simulink model "deteccion_prueba"  (R2018a)
settings: Solver=VariableStepAuto  StartTime=0.0  StopTime=0.8  RelTol=1e-3
values from neighbouring files (symbols this model uses):
  tm = 1e-4    (= 0.0001)    [SimulinkInit.m]
settings Model: Creator=cmparedes  LastModifiedBy=cmparedes

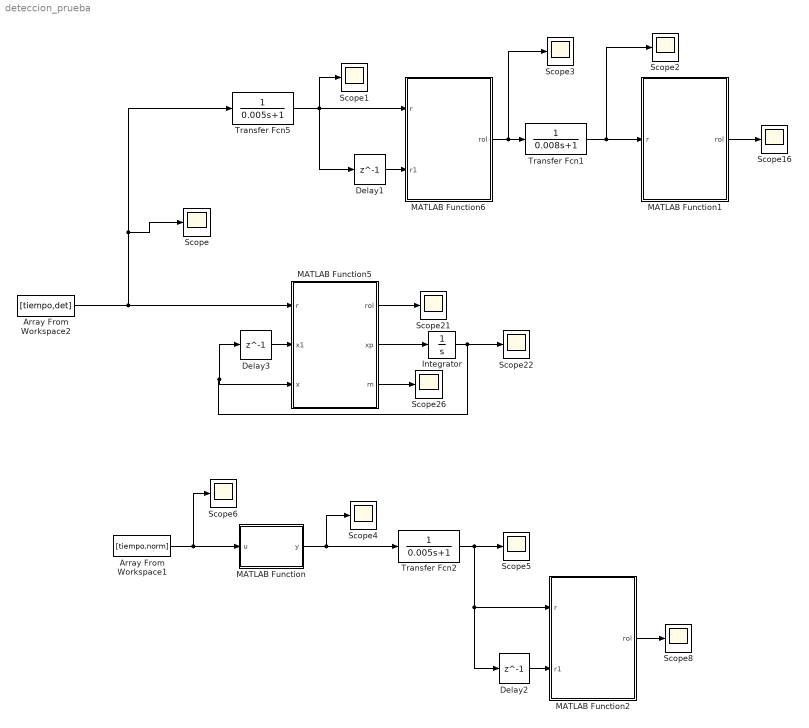
== system deteccion_prueba ==
  Array From Workspace1 : FromWorkspace  VariableName=[tiempo,norm]  SampleTime=tm
  Array From Workspace2 : FromWorkspace  VariableName=[tiempo,det]  SampleTime=tm
  Delay1 : Delay  DelayLength=1
  Delay2 : Delay  DelayLength=1
  Delay3 : Delay  DelayLength=1
  Integrator : Integrator
  MATLAB Function : MATLAB Function  TreatAsAtomicUnit=on
  MATLAB Function1 : MATLAB Function  TreatAsAtomicUnit=on
  MATLAB Function2 : MATLAB Function  TreatAsAtomicUnit=on
  MATLAB Function5 : MATLAB Function  TreatAsAtomicUnit=on
  MATLAB Function6 : MATLAB Function  TreatAsAtomicUnit=on
  Scope{,1..6,8,16,21..22,26} (12 alike) : Scope
  Transfer Fcn1 : TransferFcn  Denominator=[0.008 1]
  Transfer Fcn2 : TransferFcn  Denominator=[0.005 1]
  Transfer Fcn5 : TransferFcn  Denominator=[0.005 1]
  wires:
  MATLAB Function5/3(m) -> Scope26/1
  MATLAB Function5/1(rol) -> Scope21/1
  MATLAB Function5/2(xp) -> Integrator/1
  Integrator/1 -> Delay3/1, MATLAB Function5/3(x), Scope22/1
  MATLAB Function6/1(rol) -> Scope3/1, Transfer Fcn1/1
  Delay1/1 -> MATLAB Function6/2(r1)
  Transfer Fcn5/1 -> Scope1/1, MATLAB Function6/1(r), Delay1/1
  Array From Workspace2/1 -> Scope/1, Transfer Fcn5/1, MATLAB Function5/1(r)
  Delay3/1 -> MATLAB Function5/2(x1)
  Transfer Fcn1/1 -> Scope2/1, MATLAB Function1/1(r)
  MATLAB Function1/1(rol) -> Scope16/1
  Array From Workspace1/1 -> Scope6/1, MATLAB Function/1(u)
  Transfer Fcn2/1 -> Delay2/1, MATLAB Function2/1(r), Scope5/1
  MATLAB Function/1(y) -> Transfer Fcn2/1, Scope4/1
  Delay2/1 -> MATLAB Function2/2(r1)
  MATLAB Function2/1(rol) -> Scope8/1

== matlab function deteccion_prueba/MATLAB Function1 ==
  data: r input; rol output
function rol = fcn(r)%u1,u2,ym1,ym2)
Th_det = 6.5e-8;
% Th_det=0.1;  %2.5

if r >=Th_det
    rol=1;
else
    rol=0;
end

== matlab function deteccion_prueba/MATLAB Function ==
  data: u input; y output
function y = fcn(u)

if u>0.07

    y = 1;
else
    y=0;
end

== matlab function deteccion_prueba/MATLAB Function2 ==
  data: r input; rol output; r1 input
function rol = fcn(r,r1)%u1,u2,ym1,ym2)
Th_det = 6.5e-8;
Th_det=0.1;  %2.5

m=r-r1;
if m>0
    Th_det=0.1;  %2.5
elseif m<0 && r<=0.01
    Th_det=0.9; 
end


% sys=tf(1,[0.001 1]);


if r >=Th_det
    rol=1;
else
    rol=0;
end

== matlab function deteccion_prueba/MATLAB Function5 ==
  data: r input; rol output; x1 input; xp output; x input; m output
function [rol,xp,m]= fcn(r,x1,x)%u1,u2,ym1,ym2)
Th_det = 6.5e-8;
Th_det=0.1;  %2.5

tao1=0.002;
tao2=0.02;
m=x-x1;

xp= r/tao1-x/tao1;

% xp=0;

if m>0
    xp= r/tao1-x/tao1;
    Th_det=0.1;  %2.5
elseif m<0 && x<=-1
    xp= r/tao2-x/tao2;
    Th_det=0.08; 
end



% sys=tf(1,[0.001 1]);


if x >=Th_det
    rol=1;
else
    rol=0;
end

== matlab function deteccion_prueba/MATLAB Function6 ==
  data: r input; rol output; r1 input
function rol = fcn(r,r1)%u1,u2,ym1,ym2)
Th_det = 6.5e-8;
Th_det=0.1;  %2.5

m=r-r1;
if m>0
    Th_det=0.1;  %2.5
elseif m<0 && r<=0.01
    Th_det=0.9; 
end


% sys=tf(1,[0.001 1]);


if r >=Th_det
    rol=1;
else
    rol=0;
end
